simulink model "Ecuacion_Diferencial_Ejercicio_2"  (R2017b)
settings: Solver=ode1  StartTime=0.0  StopTime=10.0  FixedStep=0.001  RelTol=1e-3
settings Model: Creator=Elmer  LastModifiedBy=Elmer

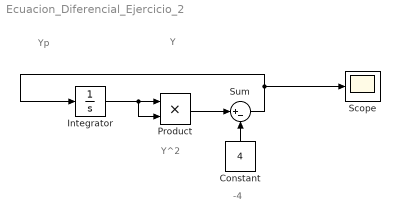
== system Ecuacion_Diferencial_Ejercicio_2 ==
  note: Y
  note: Yp
  note: Y^2
  note: -4
  Constant : Constant  Value=4
  Integrator : Integrator  InitialCondition=1
  Product : Product
  Scope : Scope
  Sum : Sum  Inputs=|+-
  wires:
  Integrator/1 -> Product/2, Product/1
  Product/1 -> Sum/1
  Constant/1 -> Sum/2
  Sum/1 -> Integrator/1, Scope/1
